simulink model "two_to_one_MUX"  (R2021a)
settings: Solver=VariableStepAuto  StartTime=0.0  StopTime=10.0  RelTol=1e-3
settings Model: Creator=kbhar  LastModifiedBy=kbhar

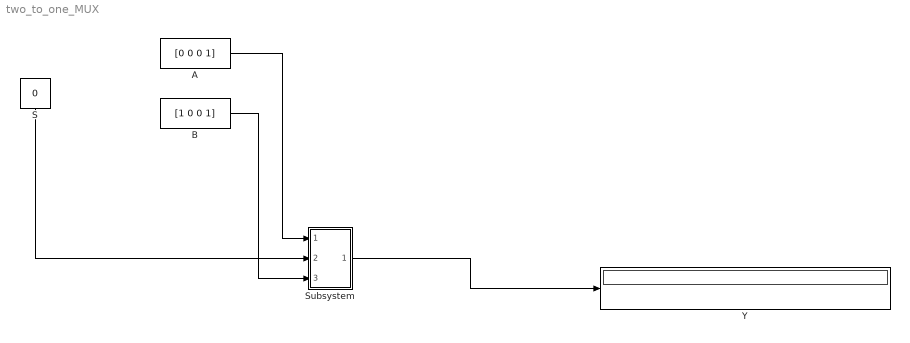
== system two_to_one_MUX ==
  A : Constant  Value=[0 0 0 1]
  B : Constant  Value=[1 0 0 1]
  S : Constant  Value=0
  Subsystem : Subsystem
  Y : Display
  wires:
  A/1 -> Subsystem/1(In_1)
  S/1 -> Subsystem/2(Sel)
  B/1 -> Subsystem/3(In_2)
  Subsystem/1(Out) -> Y/1

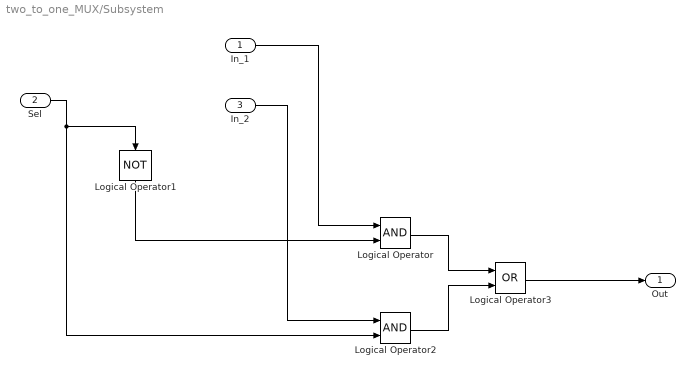
== system two_to_one_MUX/Subsystem ==
  In_1 : Inport
  Sel : Inport  Port=2
  In_2 : Inport  Port=3
  Logical Operator : Logic  AllPortsSameDT=off  OutDataTypeStr=boolean
  Logical Operator1 : Logic  Operator=NOT  AllPortsSameDT=off  OutDataTypeStr=boolean
  Logical Operator2 : Logic  AllPortsSameDT=off  OutDataTypeStr=boolean
  Logical Operator3 : Logic  Operator=OR  AllPortsSameDT=off  OutDataTypeStr=boolean
  Out : Outport
  wires:
  Logical Operator/1 -> Logical Operator3/1
  Logical Operator1/1 -> Logical Operator/2
  Sel/1 -> Logical Operator1/1, Logical Operator2/2
  Logical Operator2/1 -> Logical Operator3/2
  In_2/1 -> Logical Operator2/1
  In_1/1 -> Logical Operator/1
  Logical Operator3/1 -> Out/1
